simulink model "flightsim1"  (R2020a)
settings: Solver=VariableStepAuto  StartTime=0.0  StopTime=25  RelTol=1e-3
libraries: shared3dof x1
settings Model: Creator=jonathan  LastModifiedBy=jonathan

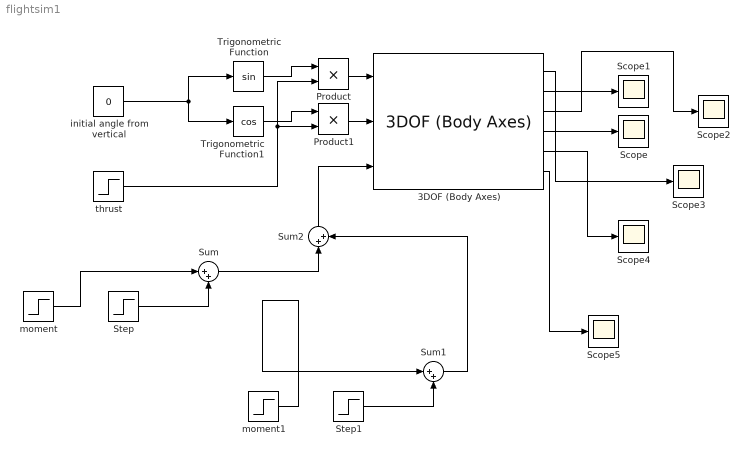
== system flightsim1 ==
  3DOF (Body Axes) : shared3dof/3DOF (Body Axes)  units=Metric (MKS)  mtype=Fixed  v_ini=0  theta_ini=0  alpha_ini=0  pos_ini=[0 0]  q_ini=0  mass=1.0  mass_e=0.5  mass_f=3.0  Iyy=1.0  Iyy_e=0.5  Iyy_f=3.0  g_in=Internal  g=-9.81  vre_flag=on  abi_flag=off  aMode=0  vel_statename=''  theta_statename=''  pos_statename=''  q_statename=''  mass_statename=''
      settings: SourceProductBaseCode=AE,PW,MT,VE,VP
  Product : Product
  Product1 : Product
  Scope{,1..5} (6 alike) : Scope
  Step : Step  Time=6  After=-0.1  SampleTime=0
  Step1 : Step  Time=10  After=0.1  SampleTime=0
  Sum : Sum  Inputs=|++
  Sum1 : Sum  Inputs=|++
  Sum2 : Sum  Inputs=|++
  Trigonometric Function : Trigonometry
  Trigonometric Function1 : Trigonometry  Operator=cos
  initial angle from vertical : Constant  Value=0
  moment : Step  Time=4  After=0.1  SampleTime=0
  moment1 : Step  Time=8  After=-0.1  SampleTime=0
  thrust : Step  Time=10  Before=15  After=0  SampleTime=0
  wires:
  3DOF (Body Axes)/4 -> Scope/1
  initial angle from vertical/1 -> Trigonometric Function1/1, Trigonometric Function/1
  Product/1 -> 3DOF (Body Axes)/1
  Product1/1 -> 3DOF (Body Axes)/2
  Trigonometric Function/1 -> Product/1
  Trigonometric Function1/1 -> Product1/1
  thrust/1 -> Product1/2, Product/2
  3DOF (Body Axes)/2 -> Scope1/1
  3DOF (Body Axes)/3 -> Scope2/1
  Step/1 -> Sum/2
  moment/1 -> Sum/1
  Sum2/1 -> 3DOF (Body Axes)/3
  3DOF (Body Axes)/1 -> Scope3/1
  Step1/1 -> Sum1/2
  moment1/1 -> Sum1/1
  Sum/1 -> Sum2/1
  Sum1/1 -> Sum2/2
  3DOF (Body Axes)/5 -> Scope4/1
  3DOF (Body Axes)/6 -> Scope5/1
